simulink model "JtrajFeed"  (R2019b)
settings: Solver=VariableStepAuto  StartTime=0.0  StopTime=10.0  RelTol=1e-3
values from neighbouring files (symbols this model uses):
  R = SerialLink(L, 'name', '210F', 'comment', 'six DOF', 'manufacturer', 'FANUC')    [Model_210F.m]    (also in Model_210F_old.m)
libraries: roblocks x5
settings Model: Creator=Karl  LastModifiedBy=Karl

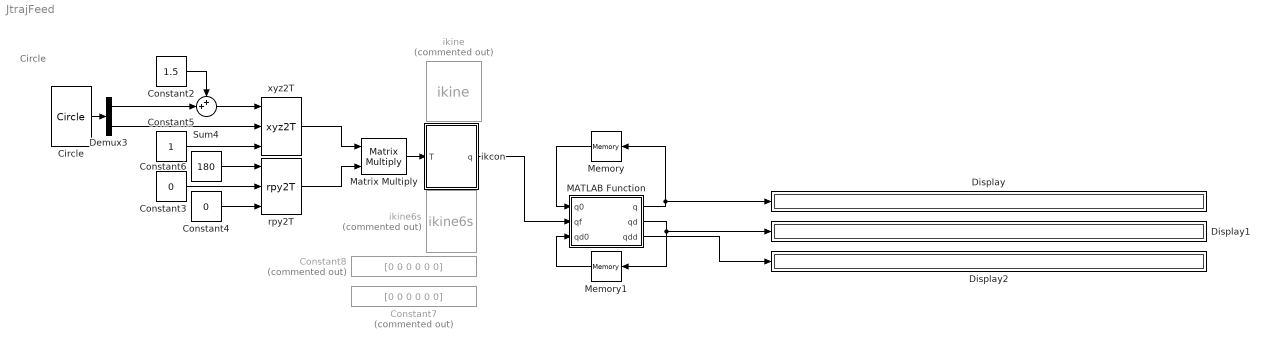
== system JtrajFeed ==
  note: Circle
  Circle : roblocks/Toolbox/Circle  radius=0.5  freq=0.1
  Constant2 : Constant  Value=1.5
  Constant3 : Constant  Value=0
  Constant4 : Constant  Value=0
  Constant5 : Constant
  Constant6 : Constant  Value=180
  Constant7 : Constant  Commented=on  Value=[0 0 0 0 0 0]
  Constant8 : Constant  Commented=on  Value=[0 0 0 0 0 0]
  Demux3 : Demux  Outputs=2
  Display : Display
  Display1 : Display
  Display2 : Display
  MATLAB Function : MATLAB Function  TreatAsAtomicUnit=on
  Matrix Multiply : Product  Multiplication=Matrix(*)
  Memory : Memory  InitialCondition=[0 0 0 0 0 0]
  Memory1 : Memory  InitialCondition=[0 0 0 0 0 0]
  Sum4 : Sum  Inputs=++|
  ikcon : Subsystem  mask{robot=R}
      mask prompts: robot "Robot object"
      mask help: Inverse kinematics for 6-axis spherical robot
      mask Help:
      | Compute joint coordinates for robot given end-effector pose.
      | 
      | 
      | <b>Parameters::</b>
      | 
      | Robot (SerialLink class)  The N-axis robot object for computing forward kinematics.
      | Configuration             Configuration string comprised of 'lrudnf'
      | 
      | <b>Inputs::</b>
      | 
      | T (4x4) the pose of the end effector as a homogeneous transformation
      | 
      | 
      | <b>Outputs::</b>
      | 
      | q (1xN) joint coordinates
      | 
      | <b>Notes::</b>
      | 
      | - A wrapper for the Toolbox method ikine6s().
  ikine : roblocks/Arm/ikine  Commented=on  robot=R.nofriction  q0=[0 -pi/4 0 0 -pi/4 0]  M=[1 1 1 1 1 1]  pinv=off  options={}
  ikine6s : roblocks/Arm/ikine6s  Commented=on  robot=R  conf='luf'
  rpy2T : roblocks/Toolbox/rpy2T  sequence=ZYX  degrees=on
  xyz2T : roblocks/Toolbox/xyz2T
  wires:
  Circle/1 -> Demux3/1
  Constant5/1 -> xyz2T/3
  Constant2/1 -> Sum4/1
  Sum4/1 -> xyz2T/1
  Constant3/1 -> rpy2T/2
  xyz2T/1 -> Matrix Multiply/1
  Demux3/1 -> Sum4/2
  Constant6/1 -> rpy2T/1
  Demux3/2 -> xyz2T/2
  Constant4/1 -> rpy2T/3
  rpy2T/1 -> Matrix Multiply/2
  ikcon/1(q) -> MATLAB Function/2(qf)
  Matrix Multiply/1 -> ikcon/1(T)
  MATLAB Function/1(q) -> Memory/1, Display/1
  MATLAB Function/2(qd) -> Memory1/1, Display1/1
  MATLAB Function/3(qdd) -> Display2/1
  Memory/1 -> MATLAB Function/1(q0)
  Memory1/1 -> MATLAB Function/3(qd0)

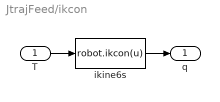
== system JtrajFeed/ikcon ==
  T : Inport
  ikine6s : MATLABFcn  MATLABFcn=robot.ikcon(u)  OutputDimensions=6
  q : Outport  VectorParamsAs1DForOutWhenUnconnected=off
  wires:
  T/1 -> ikine6s/1
  ikine6s/1 -> q/1

== matlab function JtrajFeed/MATLAB Function ==
  data: q0 input; q output; qf input; qd output; qdd output; qd0 input
function [q,qd,qdd]= fcn(q0,qf,qd0)
[q_,qd_,qdd_] = jtraj(q0, qf, 2,qd0,qd0);
q=q_(2,:);
qd=qd_(2,:);
qdd=qdd_(2,:);
end
